simulink model "unicycle_kin_trajCont_test_3"  (R2020a)
settings: Solver=FixedStepAuto  StartTime=0.0  StopTime=inf  RelTol=1e-3
undefined symbols (not defined in the file): X, Y
libraries: robotlib x5

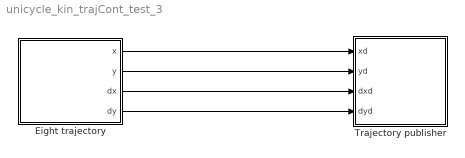
== system unicycle_kin_trajCont_test_3 ==
  Eight trajectory : Subsystem  mask{L=3, v=0.2, start=[0,0]}
      mask prompts: L "Side length"; v "Speed"; start "Start position [x, y]"
  Trajectory publisher : Subsystem  mask{simPublishRate=10}
      mask prompts: simPublishRate "Publising rate [Hz]"
  wires:
  Eight trajectory/1(x) -> Trajectory publisher/1(xd)
  Eight trajectory/2(y) -> Trajectory publisher/2(yd)
  Eight trajectory/3(dx) -> Trajectory publisher/3(dxd)
  Eight trajectory/4(dy) -> Trajectory publisher/4(dyd)

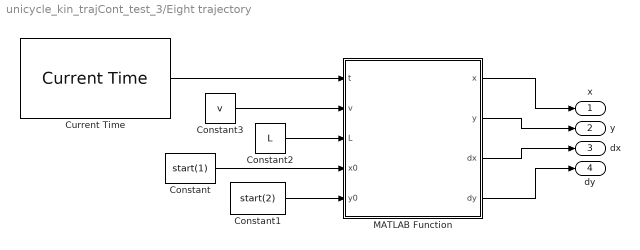
== system unicycle_kin_trajCont_test_3/Eight trajectory ==
  Constant : Constant  Value=start(1)
  Constant1 : Constant  Value=start(2)
  Constant2 : Constant  Value=L
  Constant3 : Constant  Value=v
  Current Time : robotlib/Current Time  OutputFormat=double  SampleTime=-1  ModelName=unicycle_kin_trajCont_test_3
  MATLAB Function : MATLAB Function  TreatAsAtomicUnit=on
  x : Outport
  y : Outport  Port=2
  dx : Outport  Port=3
  dy : Outport  Port=4
  wires:
  MATLAB Function/2(y) -> y/1
  Constant3/1 -> MATLAB Function/2(v)
  Constant2/1 -> MATLAB Function/3(L)
  Constant1/1 -> MATLAB Function/5(y0)
  MATLAB Function/3(dx) -> dx/1
  MATLAB Function/4(dy) -> dy/1
  Current Time/1 -> MATLAB Function/1(t)
  Constant/1 -> MATLAB Function/4(x0)
  MATLAB Function/1(x) -> x/1

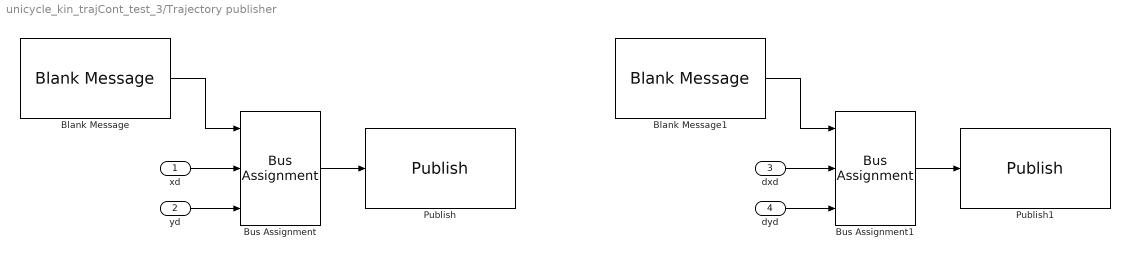
== system unicycle_kin_trajCont_test_3/Trajectory publisher ==
  xd : Inport  SampleTime=1/simPublishRate
  yd : Inport  Port=2  SampleTime=1/simPublishRate
  dxd : Inport  Port=3  SampleTime=1/simPublishRate
  dyd : Inport  Port=4  SampleTime=1/simPublishRate
  Blank Message : robotlib/Blank Message  messageClass=Message  entityType=geometry_msgs/Point  messageType=geometry_msgs/Point  SampleTime=1/simPublishRate
  Blank Message1 : robotlib/Blank Message  messageClass=Message  entityType=geometry_msgs/Point  messageType=geometry_msgs/Point  SampleTime=1/simPublishRate
  Bus Assignment : BusAssignment  AssignedSignals=X,Y
  Bus Assignment1 : BusAssignment  AssignedSignals=X,Y
  Publish : robotlib/Publish  topicSource=Specify your own  topic=/desired_position  messageType=geometry_msgs/Point  messageQueueLength=1
  Publish1 : robotlib/Publish  topicSource=Specify your own  topic=/desired_velocity  messageType=geometry_msgs/Point  messageQueueLength=1
  wires:
  Bus Assignment/1 -> Publish/1
  Blank Message/1 -> Bus Assignment/1
  xd/1 -> Bus Assignment/2
  yd/1 -> Bus Assignment/3
  dyd/1 -> Bus Assignment1/3
  dxd/1 -> Bus Assignment1/2
  Blank Message1/1 -> Bus Assignment1/1
  Bus Assignment1/1 -> Publish1/1

== matlab function unicycle_kin_trajCont_test_3/Eight trajectory/MATLAB Function ==
function [x,y,dx,dy] = eight_trajectory(t,v,L,x0,y0)
    f = 0.01;
    x = 3.0*sin(2.0*pi*t*f);
    y = 3.0*sin(4.0*pi*t*f);
    dx = 3.0*cos(2.0*pi*t*f)*2.0*pi*f;
    dy = 3.0*cos(4.0*pi*t*f)*4.0*pi*f; 
end
